simulink model "Regulacia_JCBM_Uloha2_S"  (R2022b)
settings: Solver=VariableStepAuto  StartTime=0.0  StopTime=4  RelTol=1e-8
values from neighbouring files (symbols this model uses):
  cfi = (Ua-Ra*IN)/wN    (= 2.66063720525)    [Regulacia_JCBM_M.m]
  Jc = Jm*8    (= 2.32)    [Regulacia_JCBM_M.m]
  Ki_2 = double(Ki_2)    [Regulacia_JCBM_M.m]
  Ki_5 = double(Ki_5)    [Regulacia_JCBM_M.m]
  La = 0.0081    [Regulacia_JCBM_M.m]
  Mz = MN    (= 132)    [Regulacia_JCBM_M.m]
  r1_2 = double(r1_2)    [Regulacia_JCBM_M.m]
  r1_5 = double(r1_5)    [Regulacia_JCBM_M.m]
  r2_2 = double(r2_2)    [Regulacia_JCBM_M.m]
  r2_5 = double(r2_5)    [Regulacia_JCBM_M.m]
  Ra = 0.522    [Regulacia_JCBM_M.m]
settings Model: Creator=hwswi  LastModifiedBy=hwswi

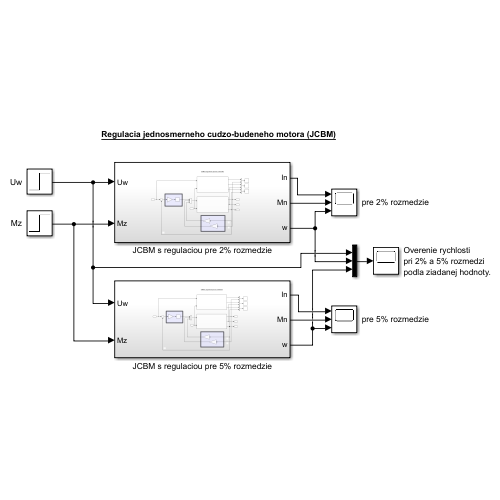
[thumbnail: Simulink's stored preview of the top-level diagram]
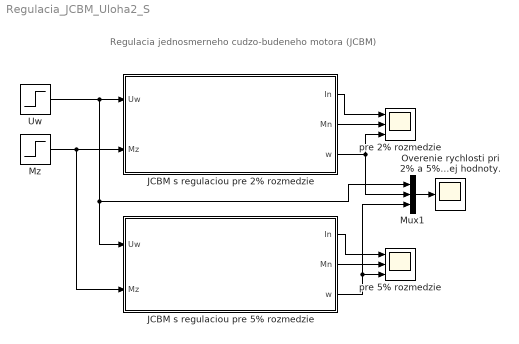
== system Regulacia_JCBM_Uloha2_S ==
  note: Regulacia jednosmerneho cudzo-budeneho motora (JCBM)
  JCBM s regulaciou pre 2% rozmedzie : Subsystem
  JCBM s regulaciou pre 5% rozmedzie : Subsystem
  Mux1 : Mux  Inputs=3
  Mz : Step  Time=2  After=Mz  SampleTime=0
  Overenie rychlosti pri 2% a 5% rozmedzi podla ziadanej hodnoty. : Scope
  Uw : Step  Time=0  After=100  SampleTime=0
  pre 2% rozmedzie : Scope  NumInputPorts=3
  pre 5% rozmedzie : Scope  NumInputPorts=3
  wires:
  JCBM s regulaciou pre 2% rozmedzie/1(In) -> pre 2% rozmedzie/1
  JCBM s regulaciou pre 2% rozmedzie/2(Mn) -> pre 2% rozmedzie/2
  Mz/1 -> JCBM s regulaciou pre 5% rozmedzie/2(Mz), JCBM s regulaciou pre 2% rozmedzie/2(Mz)
  JCBM s regulaciou pre 5% rozmedzie/2(Mn) -> pre 5% rozmedzie/2
  JCBM s regulaciou pre 5% rozmedzie/1(In) -> pre 5% rozmedzie/1
  JCBM s regulaciou pre 5% rozmedzie/3(w) -> Mux1/3, pre 5% rozmedzie/3
  JCBM s regulaciou pre 2% rozmedzie/3(w) -> Mux1/2, pre 2% rozmedzie/3
  Mux1/1 -> Overenie rychlosti pri 2% a 5% rozmedzi podla ziadanej hodnoty./1
  Uw/1 -> JCBM s regulaciou pre 5% rozmedzie/1(Uw), Mux1/1, JCBM s regulaciou pre 2% rozmedzie/1(Uw)

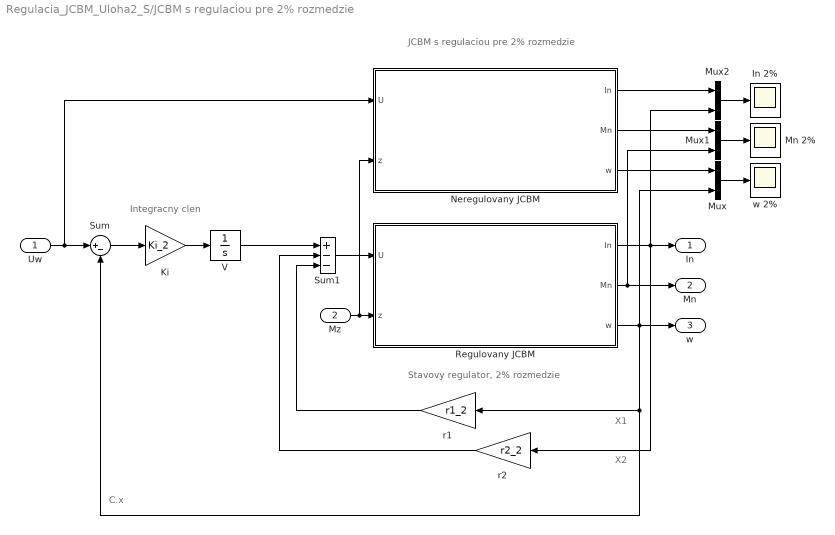
== system Regulacia_JCBM_Uloha2_S/JCBM s regulaciou pre 2% rozmedzie ==
  note: Integracny clen
  note: C.x
  note: Stavovy regulator, 2% rozmedzie
  note: JCBM s regulaciou pre 2% rozmedzie
  note: X1
  note: X2
  Uw : Inport
  Mz : Inport  Port=2
  In 2% : Scope
  Ki : Gain  Gain=Ki_2
  Mn 2% : Scope
  Mux : Mux  Inputs=2
  Mux1 : Mux  Inputs=2
  Mux2 : Mux  Inputs=2
  Neregulovany JCBM : Subsystem
  Regulovany JCBM : Subsystem
  Sum : Sum  Inputs=|+-
  Sum1 : Sum  Inputs=+--
  V : Integrator
  "r1 " : Gain  Gain=r1_2
  "r2 " : Gain  Gain=r2_2
  w 2% : Scope
  In : Outport
  Mn : Outport  Port=2
  w : Outport  Port=3
  wires:
  Regulovany JCBM/2(Mn) -> Mux1/2, Mn/1
  Mz/1 -> Neregulovany JCBM/2(z), Regulovany JCBM/2(z)
  "r1 "/1 -> Sum1/3
  Regulovany JCBM/3(w) -> Mux/2, w/1, Sum/2, "r1 "/1
  "r2 "/1 -> Sum1/2
  Mux2/1 -> In 2%/1
  Mux/1 -> w 2%/1
  Neregulovany JCBM/2(Mn) -> Mux1/1
  V/1 -> Sum1/1
  Regulovany JCBM/1(In) -> Mux2/2, "r2 "/1, In/1
  Uw/1 -> Sum/1, Neregulovany JCBM/1(U)
  Sum1/1 -> Regulovany JCBM/1(U)
  Neregulovany JCBM/3(w) -> Mux/1
  Neregulovany JCBM/1(In) -> Mux2/1
  Ki/1 -> V/1
  Mux1/1 -> Mn 2%/1
  Sum/1 -> Ki/1

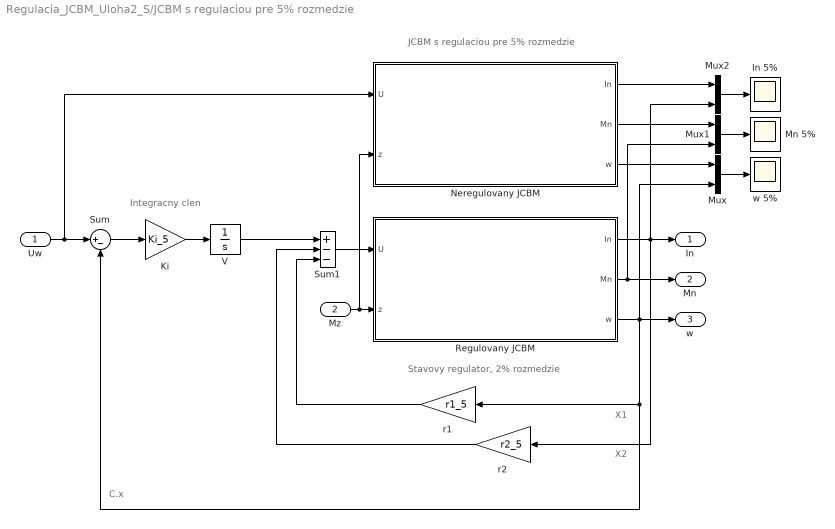
== system Regulacia_JCBM_Uloha2_S/JCBM s regulaciou pre 5% rozmedzie ==
  note: C.x
  note: X2
  note: X1
  note: Stavovy regulator, 2% rozmedzie
  note: JCBM s regulaciou pre 5% rozmedzie
  note: Integracny clen
  Uw : Inport
  Mz : Inport  Port=2
  In 5% : Scope
  Ki : Gain  Gain=Ki_5
  Mn 5% : Scope
  Mux : Mux  Inputs=2
  Mux1 : Mux  Inputs=2
  Mux2 : Mux  Inputs=2
  Neregulovany JCBM : Subsystem
  Regulovany JCBM : Subsystem
  Sum : Sum  Inputs=|+-
  Sum1 : Sum  Inputs=+--
  V : Integrator
  "r1 " : Gain  Gain=r1_5
  "r2 " : Gain  Gain=r2_5
  w 5% : Scope
  In : Outport
  Mn : Outport  Port=2
  w : Outport  Port=3
  wires:
  Ki/1 -> V/1
  Neregulovany JCBM/1(In) -> Mux2/1
  Neregulovany JCBM/3(w) -> Mux/1
  Sum1/1 -> Regulovany JCBM/1(U)
  Uw/1 -> Sum/1, Neregulovany JCBM/1(U)
  Regulovany JCBM/1(In) -> Mux2/2, "r2 "/1, In/1
  Mux1/1 -> Mn 5%/1
  Mux/1 -> w 5%/1
  V/1 -> Sum1/1
  Neregulovany JCBM/2(Mn) -> Mux1/1
  Mux2/1 -> In 5%/1
  Regulovany JCBM/3(w) -> Mux/2, w/1, Sum/2, "r1 "/1
  "r1 "/1 -> Sum1/3
  "r2 "/1 -> Sum1/2
  Mz/1 -> Neregulovany JCBM/2(z), Regulovany JCBM/2(z)
  Regulovany JCBM/2(Mn) -> Mux1/2, Mn/1
  Sum/1 -> Ki/1

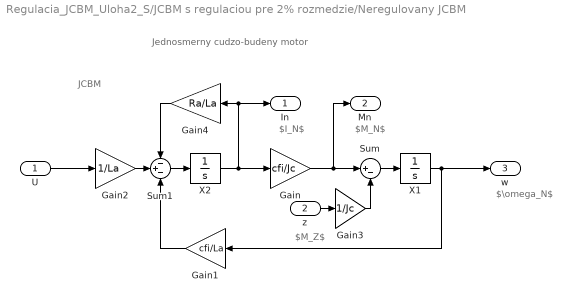
== system Regulacia_JCBM_Uloha2_S/JCBM s regulaciou pre 2% rozmedzie/Neregulovany JCBM ==
  note: JCBM
  note: Jednosmerny cudzo-budeny motor
  note: $\omega_N$
  note: $I_N$
  note: $M_N$
  note: $M_Z$
  U : Inport
  z : Inport  Port=2
  Gain : Gain  Gain=cfi/Jc
  Gain1 : Gain  Gain=cfi/La
  Gain2 : Gain  Gain=1/La
  Gain3 : Gain  Gain=1/Jc
  Gain4 : Gain  Gain=Ra/La
  Sum : Sum  Inputs=|+-
  Sum1 : Sum  Inputs=-+-
  X1 : Integrator
  X2 : Integrator
  In : Outport
  Mn : Outport  Port=2
  w : Outport  Port=3
  wires:
  X1/1 -> w/1, Gain1/1
  X2/1 -> In/1, Gain4/1, Gain/1
  Gain4/1 -> Sum1/1
  z/1 -> Gain3/1
  Gain3/1 -> Sum/2
  Gain/1 -> Mn/1, Sum/1
  Sum1/1 -> X2/1
  Gain1/1 -> Sum1/3
  Sum/1 -> X1/1
  Gain2/1 -> Sum1/2
  U/1 -> Gain2/1

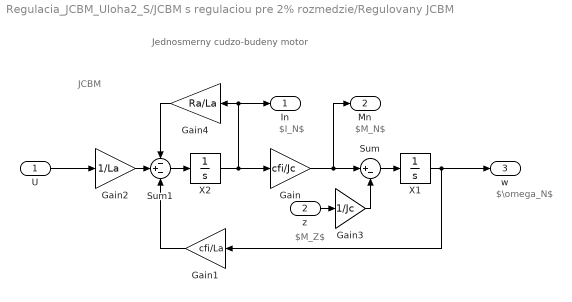
== system Regulacia_JCBM_Uloha2_S/JCBM s regulaciou pre 2% rozmedzie/Regulovany JCBM ==
  note: $M_Z$
  note: $M_N$
  note: $I_N$
  note: $\omega_N$
  note: Jednosmerny cudzo-budeny motor
  note: JCBM
  U : Inport
  z : Inport  Port=2
  Gain : Gain  Gain=cfi/Jc
  Gain1 : Gain  Gain=cfi/La
  Gain2 : Gain  Gain=1/La
  Gain3 : Gain  Gain=1/Jc
  Gain4 : Gain  Gain=Ra/La
  Sum : Sum  Inputs=|+-
  Sum1 : Sum  Inputs=-+-
  X1 : Integrator
  X2 : Integrator
  In : Outport
  Mn : Outport  Port=2
  w : Outport  Port=3
  wires:
  U/1 -> Gain2/1
  Gain2/1 -> Sum1/2
  Sum/1 -> X1/1
  Gain1/1 -> Sum1/3
  Sum1/1 -> X2/1
  Gain/1 -> Sum/1, Mn/1
  Gain3/1 -> Sum/2
  z/1 -> Gain3/1
  Gain4/1 -> Sum1/1
  X2/1 -> Gain/1, Gain4/1, In/1
  X1/1 -> Gain1/1, w/1

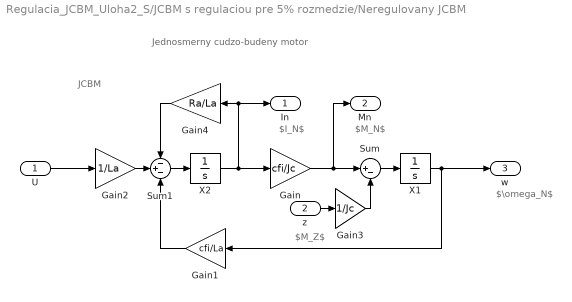
== system Regulacia_JCBM_Uloha2_S/JCBM s regulaciou pre 5% rozmedzie/Neregulovany JCBM ==
  note: JCBM
  note: Jednosmerny cudzo-budeny motor
  note: $\omega_N$
  note: $I_N$
  note: $M_N$
  note: $M_Z$
  U : Inport
  z : Inport  Port=2
  Gain : Gain  Gain=cfi/Jc
  Gain1 : Gain  Gain=cfi/La
  Gain2 : Gain  Gain=1/La
  Gain3 : Gain  Gain=1/Jc
  Gain4 : Gain  Gain=Ra/La
  Sum : Sum  Inputs=|+-
  Sum1 : Sum  Inputs=-+-
  X1 : Integrator
  X2 : Integrator
  In : Outport
  Mn : Outport  Port=2
  w : Outport  Port=3
  wires:
  X1/1 -> w/1, Gain1/1
  X2/1 -> In/1, Gain4/1, Gain/1
  Gain4/1 -> Sum1/1
  z/1 -> Gain3/1
  Gain3/1 -> Sum/2
  Gain/1 -> Mn/1, Sum/1
  Sum1/1 -> X2/1
  Gain1/1 -> Sum1/3
  Sum/1 -> X1/1
  Gain2/1 -> Sum1/2
  U/1 -> Gain2/1

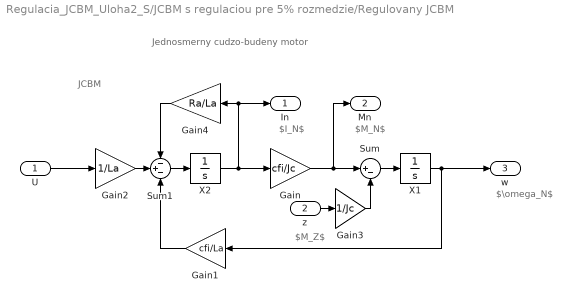
== system Regulacia_JCBM_Uloha2_S/JCBM s regulaciou pre 5% rozmedzie/Regulovany JCBM ==
  note: $M_Z$
  note: $M_N$
  note: $I_N$
  note: $\omega_N$
  note: Jednosmerny cudzo-budeny motor
  note: JCBM
  U : Inport
  z : Inport  Port=2
  Gain : Gain  Gain=cfi/Jc
  Gain1 : Gain  Gain=cfi/La
  Gain2 : Gain  Gain=1/La
  Gain3 : Gain  Gain=1/Jc
  Gain4 : Gain  Gain=Ra/La
  Sum : Sum  Inputs=|+-
  Sum1 : Sum  Inputs=-+-
  X1 : Integrator
  X2 : Integrator
  In : Outport
  Mn : Outport  Port=2
  w : Outport  Port=3
  wires:
  U/1 -> Gain2/1
  Gain2/1 -> Sum1/2
  Sum/1 -> X1/1
  Gain1/1 -> Sum1/3
  Sum1/1 -> X2/1
  Gain/1 -> Sum/1, Mn/1
  Gain3/1 -> Sum/2
  z/1 -> Gain3/1
  Gain4/1 -> Sum1/1
  X2/1 -> Gain/1, Gain4/1, In/1
  X1/1 -> Gain1/1, w/1
